simulink library "qss_tb_library_aalto"  (Simulink 8.3)
settings: Solver=ode45  SolverMode=SingleTasking  StartTime=0.0  StopTime=1220  RelTol=1e-3
undefined symbols (not defined in the file): c_BT_E1, c_BT_E2, c_BT_E3, c_BT_E4, c_BT_L1, c_BT_L2, c_BT_L3, c_BT_L4, cap_BT, cc_done, delta_h_C_air, DiscIntNeverNeededParam, dw_GG_c, eff_FC_max, eta_EG_map, eta_EM_map, g, h, H_o_m, H_u, I_BT_max, i_FC_in, i_FC_max, k1, k2, k3, k4, k_cs, M_air, manual_gearbox, P_CVT_opt, power_max, Q_BT_0, Q_BT_IC, Q_BT_min, Q_SC_IC, r_wheel, rchg_map_BT, rdis_map_BT, rho, rho_f, soc_map_BT, t_c, T_CE_max, T_EG_c, T_EG_max, T_EM_max, T_z, U_BT_0, V, V_CE_map, V_FC_out, voc_map_BT, w_CE_max, w_CE_upper, w_CVT_opt, w_EG_row, w_EG_upper, w_EM_row, w_EM_upper ... (+1)
libraries: simulink x4
(part 1 of 4)
settings Model: Creator=buehli  LastModifiedBy=alajunen  ExtModeAutoUpdateStatusClock=off

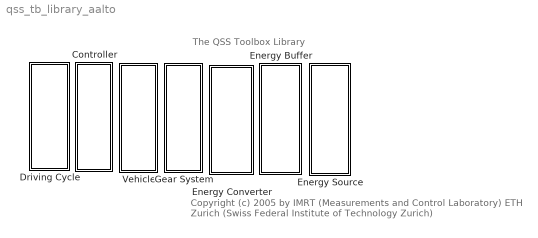
== system qss_tb_library_aalto ==
  note: Copyright (c) 2005 by IMRT (Measurements and Control Laboratory)
      | ETH Zurich (Swiss Federal Institute of Technology Zurich)
  note: The QSS Toolbox Library
  Controller : Subsystem
      mask Display: disp('Controller')
  Driving Cycle : Subsystem
      mask Display: disp('Driving Cycle')
  Energy Buffer : Subsystem
      mask Display: disp('Energy Buffer')
  Energy Converter : Subsystem
      mask Display: disp('Energy Converter')
  Energy Source : Subsystem
      mask Display: disp('Energy Source')
  Gear System : Subsystem
      mask Display: disp('Gear System')
  Vehicle : Subsystem
      mask Display: disp('Vehicle')

== system qss_tb_library_aalto/Controller ==
  Battery Controller : Subsystem  mask(Battery Controller){}
      mask help:
      | Control strategy (very primitive):
      | ========================
      | As soon as battery charge drops below level Q_BT_min, the CE/Generator
      | are started and operated at given load/speed for a fixed time period.
      | This time has been selected to guarantee the same battery level at the
      | end of the cycle.
      mask init:
      | init_BT_ctrl;
  CVT Controller : Subsystem  Tag=cvt controller  mask(CVT Controller){j_CVT_min=3, j_CVT_max=15, w_wheel_min=3, w_CVT_idle=100, w_CVT_upper=300}
      mask prompts: j_CVT_min "Lower gear ratio limit [-]"; j_CVT_max "Upper gear ratio limit [-]"; w_wheel_min "Minimum wheel speed [rad/s]"; w_CVT_idle "CVT idle speed [rad/s]"; w_CVT_upper "Maximum CVT speed [rad/s]"
      mask help:
      | This block calculates the optimum gear ratio and its change during one integration step for a CVT.
      |
      | Input:
      | =====
      | 	v		Speed [m/s]
      | 	dv		Acceleration [m/s^2]
      |
      | Output:
      | ======
      | 	v_delay		Speed one step delayed [m/s]
      | 	dv_delay	Acceleration one step delayed [m/s^2]
      | 	j_CVT		Gear ratio [-]
      | 	dj_CVT		Change of gear ratio [1/s]
      mask init:
      | init_CVT_ctrl;
  Control Unit (empty template) : Subsystem  Tag=control unit  mask(Control Unit){}
      mask help:
      | This block gives the user the opportunity to design his/her own control unit.
      |
      | The user can define the inputs and outputs  by himself/herself.
  Gen-set Controller v2 : Subsystem  mask(Engine-Generator Controller){}
      mask help:
      | Control strategy description:
      | ==============================
      | This block controls the use of the Engine-Generator set (Gen-set).
      | The control system has two different parts: Engine start up/shut down control,
      | and the control of Gen-set power when running.
      |
      | The Engine start up/shut down and Gen-set power are controller by simple rules
      | based on:
      | * vehicle speed, and
      | * battery state-of-charge (soc)
      |
      | The parameters for the Engine start up/shut down control are given in the mask
      | of the block. The parameters for the Gen-set power control are defined in the
      | Look-up tables and the reference control speed is given through the block mask.
      mask init:
      | global h
  Gen-set Controller : Subsystem  mask(Engine-Generator Controller){}
      mask help:
      | Control strategy description:
      | ==============================
      | This block controls the use of the Engine-Generator set (Gen-set).
      | The control system has two different parts: Engine start up/shut down control,
      | and the control of Gen-set power when running.
      |
      | The Engine start up/shut down and Gen-set power are controller by simple rules
      | based on:
      | * vehicle speed, and
      | * battery state-of-charge (soc)
      |
      | The parameters for the Engine start up/shut down control are given in the mask
      | of the block. The parameters for the Gen-set power control are defined in the
      | Look-up tables and the reference control speed is given through the block mask.
      mask init:
      | global h

== system qss_tb_library_aalto/Driving Cycle ==
  Driving Cycle : Subsystem  Tag=cycle  mask(Driving Cycle){cyclenr=Europe: NEDC, stepsize=1, autostop=on}
      mask prompts: cyclenr "Choose a cycle"; stepsize "Step size [s]"; autostop "Enable automatic simulation stop"
      mask help:
      | This block loads the cycle data such as time, speed, acceleration and gear number,  from the specified data file and makes it available on the output of the cycle block.
      |
      | Output:
      | ======
      | 	v	Speed [m/s]
      | 	dv	Acceleration [m/s^2]
      | 	i	Gear number [-]
      | 	x_tot	Total distance [m]
      |
      | Tip:
      | ===
      | Probably you don't need the gear number "i". If so you can terminate
      | it with a "Terminator" out of the "Simulink Library/Connections."
      |
      | Step size:
      | ========
      | Default value is 1. Don't change it, unless you are familiar with the programs of the QSS TB.
      |
      | Enable automatic simulation stop:
      | ===========================
      | Stops the simulation automatically at the end of the cycle.
      | Be careful: If you have a component in your model that has to run after the cycle has finished, e.g. a battery to charge, remove the mark!
      mask init:
      | init_driving_cycle;
      mask TypeOptions cyclenr: Europe: ECE manual | Europe: ECE R15 spez | Europe: ECE R15 | Europe: EUDC | Europe: EUDC manual | Europe: City | Europe: City manual | Europe: NEDC | Europe: NEDC manual | Japan:  10-15-Mode | Japan:  10-Mode | Japan:  10-Mode-3 | Japan:  11-Mode | Japan:  11-Mode-4 | Japan:  15-Mode | USA:    City-I | USA:    City-II | USA:    FTP-75 | USA:    FTP-Highway
      mask Display: plot(T_zplot, V_zplot);
  Driving Cycle v2 : Subsystem  Tag=cycle  mask(Driving Cycle){cyclenr=Europe: NEDC, stepsize=1, autostop=on}
      mask prompts: cyclenr "Choose a cycle"; stepsize "Step size [s]"; autostop "Enable automatic simulation stop"
      mask help:
      | This block loads the cycle data such as time, speed, acceleration and gear number,  from the specified data file and makes it available on the output of the cycle block.
      |
      | Output:
      | ======
      | 	v	Speed [m/s]
      | 	dv	Acceleration [m/s^2]
      | 	i	Gear number [-]
      | 	x_tot	Total distance [m]
      |
      | Tip:
      | ===
      | Probably you don't need the gear number "i". If so you can terminate
      | it with a "Terminator" out of the "Simulink Library/Connections."
      |
      | Step size:
      | ========
      | Default value is 1. Don't change it, unless you are familiar with the programs of the QSS TB.
      |
      | Enable automatic simulation stop:
      | ===========================
      | Stops the simulation automatically at the end of the cycle.
      | Be careful: If you have a component in your model that has to run after the cycle has finished, e.g. a battery to charge, remove the mark!
      mask init:
      | init_driving_cycle_v2;
      mask TypeOptions cyclenr: Europe: ECE manual | Europe: ECE R15 spez | Europe: ECE R15 | Europe: EUDC | Europe: EUDC manual | Europe: City | Europe: City manual | Europe: NEDC | Europe: NEDC manual | Japan:  10-15-Mode | Japan:  10-Mode | Japan:  10-Mode-3 | Japan:  11-Mode | Japan:  11-Mode-4 | Japan:  15-Mode | USA:    City-I | USA:    City-II | USA:    FTP-75 | USA:    FTP-Highway | USA:    US06 | USA:    SC03
      mask Display: plot(T_zplot, V_zplot);
  Driving Cycle v3 : Subsystem  Tag=cycle  mask(Driving Cycle){cyclenr=Europe: NEDC, stepsize=1, autostop=on}
      mask prompts: cyclenr "Choose a cycle"; stepsize "Step size [s]"; autostop "Enable automatic simulation stop"
      mask help:
      | This block loads the cycle data such as time, speed, acceleration and gear number,  from the specified data file and makes it available on the output of the cycle block.
      |
      | Output:
      | ======
      | 	v	Speed [m/s]
      | 	dv	Acceleration [m/s^2]
      | 	i	Gear number [-]
      | 	x_tot	Total distance [m]
      |
      | Tip:
      | ===
      | Probably you don't need the gear number "i". If so you can terminate
      | it with a "Terminator" out of the "Simulink Library/Connections."
      |
      | Step size:
      | ========
      | Default value is 1. Don't change it, unless you are familiar with the programs of the QSS TB.
      |
      | Enable automatic simulation stop:
      | ===========================
      | Stops the simulation automatically at the end of the cycle.
      | Be careful: If you have a component in your model that has to run after the cycle has finished, e.g. a battery to charge, remove the mark!
      mask init:
      | init_driving_cycle_v3;
      mask TypeOptions cyclenr: Europe: ECE manual | Europe: ECE R15 spez | Europe: ECE R15 | Europe: EUDC | Europe: EUDC manual | Europe: City | Europe: City manual | Europe: NEDC | Europe: NEDC manual | Japan:  10-15-Mode | Japan:  10-Mode | Japan:  10-Mode-3 | Japan:  11-Mode | Japan:  11-Mode-4 | Japan:  15-Mode | Japan:  JC08 | USA:    City-I | USA:    City-II | USA:    FTP-75 | USA:    FTP-Highway | USA:    US06 | USA:    SC03 | World:  WLTC
      mask Display: plot(T_zplot, V_zplot);

== system qss_tb_library_aalto/Energy Buffer ==
  Battery : Subsystem  Tag=battery  mask(Battery){I_0=100, Q_BT_IC_rel=27.78, t_ch=20}
      mask prompts: I_0 "Energy capacity of battery [Ah]"; Q_BT_IC_rel "Initial charge of battery [%]"; t_ch "Current limit: minimum time to charge/discharge the battery [min]"
      mask help:
      | This block simulates a battery.
      | The resistance depends on the charge state and the charge/discharge current of the battery. The battery has an open circuit voltage of 130 V (fully charged).
      |
      | Input:
      | =====
      | 	x_tot	Total distance [m]
      | 	P_BT	Power from/to the battery [W]
      | 		P_BT < 0: battery charging
      | 		P_BT > 0: battery discharging
      |
      | Output:
      | ======
      | 	Q_BT	Current charge of the battery [C]
      | 	V_BT	Energy consumption [kWh/100 km]
      mask init:
      | init_BT;
  Battery v2 : Subsystem  Tag=battery  mask(Battery){init_soc_BT=0.7, cell_series_BT=70, cell_parallel_BT=1, init_file_BT='init_Saft_BT'}
      mask prompts: init_soc_BT "Initial charge of battery"; cell_series_BT "Cells in series"; cell_parallel_BT "Cells in parallel"; init_file_BT "Battery initialization file"
      mask init:
      | eval(init_file_BT)
  Battery v3 : Subsystem  Tag=battery  mask(Battery){init_soc_BT=0.7, cell_series_BT=70, cell_parallel_BT=1, init_file_BT='init_Saft_BT'}
      mask prompts: init_soc_BT "Initial charge of battery"; cell_series_BT "Cells in series"; cell_parallel_BT "Cells in parallel"; init_file_BT "Battery initialization file"
      mask init:
      | eval(init_file_BT)
  Supercapacitor : Subsystem  Tag=supercap  mask(Supercapacitor){C_SC=8, R_SC=0.72, U_SC_max=225, P_SC_max=17500, Q_SC_IC_rel=95, N_SC=6}
      mask prompts: C_SC "Capacity of each supercap [F]"; R_SC "Internal resistance of each supercap [Ohm]"; U_SC_max "Maximum voltage of each supercap  [V]"; P_SC_max "Maximum power of each supercap [W]"; Q_SC_IC_rel "Initial charge of each supercap [%]"; N_SC "Number of supercaps (parallel connection) [-]"
      mask help:
      | The supercap is a fast electric energy buffer.
      |
      | Input:
      | =====
      | 	P_SC	Power to/from the supercap [W]
      | 		P_SC < 0: SC charging
      | 		P_SC > 0: SC discharging
      |
      | Output:
      | ======
      | 	U_SC	Voltage of the supercap [V]
      mask init:
      | init_SC;
  Supercapacitor v2 : Subsystem  Tag=supercap  mask(Supercapacitor){C_SC=8, R_SC=0.72, U_SC_max=225, P_SC_max=17500, Q_SC_IC_rel=90, N_SC=6}
      mask prompts: C_SC "Capacity of each supercap [F]"; R_SC "Internal resistance of each supercap [Ohm]"; U_SC_max "Maximum voltage of each supercap  [V]"; P_SC_max "Maximum power of each supercap [W]"; Q_SC_IC_rel "Initial charge of each supercap [%]"; N_SC "Number of supercaps (parallel connection) [-]"
      mask help:
      | The supercap is a fast electric energy buffer.
      |
      | Input:
      | =====
      | 	P_SC	Power to/from the supercap [W]
      | 		P_SC < 0: SC charging
      | 		P_SC > 0: SC discharging
      |
      | Output:
      | ======
      | 	U_SC	Voltage of the supercap [V]
      mask init:
      | init_SC_hyb;
  Supercapacitor v3 : Subsystem  Tag=supercap  mask(Supercapacitor){C_SC=8, R_SC=0.72, U_SC_max=225, P_SC_max=17500, Q_SC_IC_rel=80, N_SC=6}
      mask prompts: C_SC "Capacity of each supercap [F]"; R_SC "Internal resistance of each supercap [Ohm]"; U_SC_max "Maximum voltage of each supercap  [V]"; P_SC_max "Maximum power of each supercap [W]"; Q_SC_IC_rel "Initial charge of each supercap [%]"; N_SC "Number of supercaps (parallel connection) [-]"
      mask help:
      | The supercap is a fast electric energy buffer.
      |
      | Input:
      | =====
      | 	P_SC	Power to/from the supercap [W]
      | 		P_SC < 0: SC charging
      | 		P_SC > 0: SC discharging
      |
      | Output:
      | ======
      | 	U_SC	Voltage of the supercap [V]
      mask init:
      | init_SC_hyb_v2;

== system qss_tb_library_aalto/Energy Converter ==
  Combustion Engine (Willans-approximation) : Subsystem  Tag=combustion engine  mask(Combustion Engine (based on Willans approximation)){engine_type=Otto, V_d=0.708, theta_CE=0.05, S=50, B=45, w_CE_idle=105, P_CE_idle=2600, P_aux=300, e=0.46, PI=2, p_me0g=1, ENABLE_FUEL_CUTOFF=on, T_CE_cutoff=5, P_CE_cutoff=0}
      mask prompts: engine_type "Engine type"; V_d "Displacement [l]"; theta_CE "Engine inertia [kg*m^2]"; S "Stroke [mm]"; B "Bore diameter [mm]"; w_CE_idle "Engine speed at idle [rad/s]"; P_CE_idle "Engine power at idle [W]"; P_aux "Power required by auxiliaries  [W]"; e "1. Willans parameter: Engine internal thermodynamic efficiency [-]"; PI "2. Willans parameter: Maximum boost ratio [-]"; p_me0g "3. Willans parameter: Gas exchange losses [bar]"; ENABLE_FUEL_CUTOFF "Enable fuel cutoff"; T_CE_cutoff "Engine torque at fuel cutoff [Nm]"; P_CE_cutoff "Power at fuel cutoff [W]"
      mask help:
      | This block simulates the behaviour of a combustion engine. The block is based on the Willans approximation with friction part based on the ETH model.
      |
      | Input:
      | =====
      | 	w_gear		Speed of the fly wheel [rad/s]
      | 	dw_gear	Acceleration of the fly wheel [rad/s^2]
      | 	T_gear		Torque on the fly wheel [Nm]
      |
      | Output:
      | ======
      | 	P_CE		Power produced by the combustion engine [W]
      mask init:
      | init_CE_willans;
      mask TypeOptions engine_type: Otto | Diesel
  Combustion Engine (consumption map) : Subsystem  Tag=combustion engine  mask(Combustion Engine (based on consumption map)){engine_type=Otto, V_d=0.708, scale_CE=1, theta_CE=0.05, w_CE_idle=105, P_CE_idle=2600, P_aux=300, ENABLE_FUEL_CUTOFF=on, T_CE_cutoff=5, P_CE_cutoff=0}
      mask prompts: engine_type "Engine type"; V_d "Displacement [l]"; scale_CE "Engine scaling factor [-]"; theta_CE "Engine inertia [kg*m^2]"; w_CE_idle "Engine speed at idle [rad/s]"; P_CE_idle "Engine power at idle [W]"; P_aux "Power required by auxiliaries [W]"; ENABLE_FUEL_CUTOFF "Enable fuel cutoff"; T_CE_cutoff "Engine torque at fuel cutoff [Nm]"; P_CE_cutoff "Power at fuel cutoff [W]"
      mask help:
      | This block simulates the behaviour of a combustion engine. The block is based on a consumption map.
      |
      | Input:
      | =====
      | 	w_gear		Speed of the fly wheel [rad/s]
      | 	dw_gear	Acceleration of the fly wheel [rad/s^2]
      | 	T_gear		Torque on the fly wheel [Nm]
      |
      | Output:
      | ======
      | 	P_CE		Power produced by the combustion engine [W]
      mask init:
      | init_CE_map;
      mask TypeOptions engine_type: Otto | Diesel
  Combustion Engine (hybrid vehicle) : Subsystem  Tag=combustion engine  mask(Combustion Engine (based on consumption map)){engine_type=Otto, V_d=1.0, theta_CE=0.05, w_CE_idle=105, P_CE_idle=0, P_aux=0, ENABLE_FUEL_CUTOFF=on, T_CE_cutoff=0, P_CE_cutoff=0}
      mask prompts: engine_type "Engine type"; V_d "Displacement [l]"; theta_CE "Engine inertia [kg*m^2]"; w_CE_idle "Engine speed at idle [rad/s]"; P_CE_idle "Engine power at idle [W]"; P_aux "Power required by auxiliaries [W]"; ENABLE_FUEL_CUTOFF "Enable fuel cutoff"; T_CE_cutoff "Engine torque at fuel cutoff [Nm]"; P_CE_cutoff "Power at fuel cutoff [W]"
      mask help:
      | This block simulates the behaviour of a combustion engine. The block is based on a consumption map.
      |
      | Input:
      | =====
      | 	w_gear		Speed of the fly wheel [rad/s]
      | 	dw_gear	Acceleration of the fly wheel [rad/s^2]
      | 	T_gear		Torque on the fly wheel [Nm]
      |
      | Output:
      | ======
      | 	P_CE		Power produced by the combustion engine [W]
      mask init:
      | init_CE_hyb_map;
      mask TypeOptions engine_type: Otto
  Combustion Engine (hybrid vehicle) v2 : Subsystem  Tag=combustion engine  mask(Combustion Engine (based on consumption map)){engine_type=Otto, V_d=V, theta_CE=0.16, w_CE_idle=105, P_CE_idle=0, P_aux=0, ENABLE_FUEL_CUTOFF=on, T_CE_cutoff=0, P_CE_cutoff=0}
      mask prompts: engine_type "Engine type"; V_d "Displacement [l]"; theta_CE "Engine inertia [kg*m^2]"; w_CE_idle "Engine speed at idle [rad/s]"; P_CE_idle "Engine power at idle [W]"; P_aux "Power required by auxiliaries [W]"; ENABLE_FUEL_CUTOFF "Enable fuel cutoff"; T_CE_cutoff "Engine torque at fuel cutoff [Nm]"; P_CE_cutoff "Power at fuel cutoff [W]"
      mask help:
      | This block simulates the behaviour of a combustion engine. The block is based on a consumption map.
      |
      | Input:
      | =====
      | w_gear	Speed of the fly wheel [rad/s]
      | dw_gear	Acceleration of the fly wheel [rad/s^2]
      | T_gear	Torque on the fly wheel [Nm]
      |
      | Output:
      | ======
      | P_CE	Power produced by the combustion engine [W]
      mask init:
      | init_CE_Prius_map;
      mask TypeOptions engine_type: Otto
  Combustion Engine v2 : Subsystem  Tag=combustion engine  mask(Combustion Engine (based on consumption map)){engine_type=Otto, V_d=1.9, theta_CE=0.1, w_CE_idle=105, P_CE_idle=2600, P_aux=300, ENABLE_FUEL_CUTOFF=on, T_CE_cutoff=5, P_CE_cutoff=0}
      mask prompts: engine_type "Engine type"; V_d "Displacement [l]"; theta_CE "Engine inertia [kg*m^2]"; w_CE_idle "Engine speed at idle [rad/s]"; P_CE_idle "Engine power at idle [W]"; P_aux "Power required by auxiliaries [W]"; ENABLE_FUEL_CUTOFF "Enable fuel cutoff"; T_CE_cutoff "Engine torque at fuel cutoff [Nm]"; P_CE_cutoff "Power at fuel cutoff [W]"
      mask help:
      | This block simulates the behaviour of a combustion engine. The block is based on a consumption map.
      |
      | Input:
      | =====
      | 	w_gear		Speed of the fly wheel [rad/s]
      | 	dw_gear	Acceleration of the fly wheel [rad/s^2]
      | 	T_gear		Torque on the fly wheel [Nm]
      |
      | Output:
      | ======
      | 	P_CE		Power produced by the combustion engine [W]
      mask init:
      | % Spark ignited (SI)
      | if engine_type == 1
      |     init_SI_CE_map;
      | end
      | % Compression ignited (CI)
      | if engine_type == 2
      |     init_CI_CE_map;
      | end
      mask TypeOptions engine_type: Otto | Diesel
  Combustion Engine v3 : Subsystem  Tag=combustion engine  mask(Combustion Engine (based on consumption map)){engine_type=Otto, V_d=1.9, theta_CE=0.1, w_CE_idle=105, P_CE_idle=0, P_aux=300, ENABLE_FUEL_CUTOFF=on, T_CE_cutoff=2, P_CE_cutoff=0}
      mask prompts: engine_type "Engine type"; V_d "Displacement [l]"; theta_CE "Engine inertia [kg*m^2]"; w_CE_idle "Engine speed at idle [rad/s]"; P_CE_idle "Engine power at idle [W]"; P_aux "Power required by auxiliaries [W]"; ENABLE_FUEL_CUTOFF "Enable fuel cutoff"; T_CE_cutoff "Engine torque at fuel cutoff [Nm]"; P_CE_cutoff "Power at fuel cutoff [W]"
      mask help:
      | This block simulates the behaviour of a combustion engine. The block is based on a consumption map.
      |
      | Input:
      | =====
      | w_gear	Speed of the fly wheel [rad/s]
      | dw_gear	Acceleration of the fly wheel [rad/s^2]
      | T_gear	Torque on the fly wheel [Nm]
      |
      | Output:
      | ======
      | P_CE	Power produced by the combustion engine [W]
      mask init:
      | % Spark ignited (SI)
      | if engine_type == 1
      |     init_SI_CE_map_v2;
      | end
      | % Compression ignited (CI)
      | if engine_type == 2
      |     init_CI_CE_map_v2;
      | end
      mask TypeOptions engine_type: Otto | Diesel
  Electric Generator : Subsystem  mask(Electric Generator){scale_EG=1}
      mask prompts: scale_EG "Generator scaling factor [-]"
      mask help:
      | This block simulates the behaviour of an electric generator. The block is based on an efficiency map.
      |
      | Input:
      | =====
      | 	w_gear		Speed of the fly wheel [rad/s]
      | 	T_gear		Torque on the fly wheel [Nm]
      |
      | Output:
      | ======
      | 	P_EG		Power of the electric generator [W]
      mask init:
      | init_EG;
  Electric Generator v2 : Subsystem  mask(Electric Generator){}
      mask help:
      | This block simulates the behaviour of an electric generator. The block is based on an efficiency map.
      |
      | Input:
      | =====
      | 	w_gear		Speed of the fly wheel [rad/s]
      | 	T_gear		Torque on the fly wheel [Nm]
      |
      | Output:
      | ======
      | 	P_EG		Power of the electric generator [W]
      mask init:
      | init_EG_hyb;
  Electric Generator v3 : Subsystem  mask(Electric Generator){init_file_name='init_EG_UQM'}
      mask prompts: init_file_name "Initialization file name"
      mask help:
      | This block simulates the behaviour of an electric generator. The block is based on an efficiency map.
      |
      | Input:
      | =====
      | w_gear		Speed of the transmission [rad/s]
      | T_gear		Torque of the transmission [Nm]
      |
      | Output:
      | ======
      | P_EG		Power of the electric generator [W]
      mask init:
      | eval(init_file_name);
  Electric Motor : Subsystem  mask(Electric Motor){scale_EM=1, theta_EM=0.1, P_aux=0}
      mask prompts: scale_EM "Motor scaling factor [-]"; theta_EM "Motor inertia [kg*m2]"; P_aux "Power required by auxiliaries [W]"
      mask help:
      | This block simulates the behaviour of an electric motor. The block is based on an efficiency map.
      |
      | Input:
      | =====
      | 	w_gear		Speed of the fly wheel [rad/s]
      | 	dw_gear	Acceleration of the fly wheel [rad/s^2]
      | 	T_gear		Torque on the fly wheel [Nm]
      |
      | Output:
      | ======
      | 	P_EM		Power produced by the electric motor [W]
      mask init:
      | init_EM;
  Electric Motor v2 : Subsystem  mask(Electric Motor){scale_EM=3.5, theta_EM=0.1, P_aux=300, over_factor=1.25}
      mask prompts: scale_EM "Motor scaling factor [-]"; theta_EM "Motor inertia [kg*m2]"; P_aux "Power required by auxiliaries [W]"; over_factor "Overtorque factor"
      mask help:
      | This block simulates the behaviour of an electric motor. The block is based on an efficiency map.
      |
      | Input:
      | =====
      | 	w_gear		Speed of the fly wheel [rad/s]
      | 	dw_gear	Acceleration of the fly wheel [rad/s^2]
      | 	T_gear		Torque on the fly wheel [Nm]
      |
      | Output:
      | ======
      | 	P_EM		Power produced by the electric motor [W]
      mask init:
      | init_EM;
  Fuel Cell : Subsystem  Tag=fuelcell  mask(Fuel Cell){N_FC=880, A_FC=190 * 1e4, V_th=1.2, P_FC_idle=2000, eta_EM_C=0.75, eta_C=0.7, pi_C=1.3, T_air=25, l_air=1.5}
      mask prompts: N_FC "Number of fuel cells per stack (series connection) [-]"; A_FC "Size of fuel cell [m^2]"; V_th "Theoretical fuel cell voltage [V]"; P_FC_idle "Idle power [W]"; eta_EM_C "E-motor for air compressor efficiency [-]"; eta_C "Air compressor efficiency [-]"; pi_C "Air compression ratio [-]"; T_air "Air temperature [°C]"; l_air "Air to fuel ratio [-]"
      mask help:
      | This block simulates a fuel cell and converts fuel into electric energy.
      |
      | Input:
      | =====
      | 	P_in		Power required by the fuel cell [W]
      |
      | Output:
      | ======
      | 	P_FC		Power produced by the fuel cell [W]
      mask init:
      | init_FC;
  Fuel Cell v2 : Subsystem  Tag=fuelcell  mask(Fuel Cell){N_FC=120, A_FC=0.084, V_th=1.2, P_FC_idle=2000, eta_EM_C=0.75, eta_C=0.7, pi_C=1.3, T_air=25, l_air=1.5}
      mask prompts: N_FC "Number of fuel cells per stack (series connection) [-]"; A_FC "Size of a single fuel cell [m^2]"; V_th "Theoretical fuel cell voltage [V]"; P_FC_idle "Idle power [W]"; eta_EM_C "E-motor for air compressor efficiency [-]"; eta_C "Air compressor efficiency [-]"; pi_C "Air compression ratio [-]"; T_air "Air temperature [°C]"; l_air "Air to fuel ratio [-]"
      mask help:
      | This block simulates a fuel cell and converts fuel into electric energy.
      |
      | Input:
      | =====
      | 	P_in		Power required by the fuel cell [W]
      |
      | Output:
      | ======
      | 	P_FC		Power produced by the fuel cell [W]
      mask init:
      | init_FC_hyb;

== system qss_tb_library_aalto/Energy Source ==
  Display : Display
  Hydrogen Tank : Subsystem  Tag=tank  mask(Tank){flag_cold_start=off}
      mask prompts: flag_cold_start "Include cold start losses"
      mask help:
      | This block integrates the power (the fuel mass flow) required by the combustion engine or the fuel cell and calculates the energy consumption in liter/100 km.
      |
      | Input:
      | =====
      | 	P_fuel	Power (fuel mass flow) required [W]
      | 	x_tot	Total distance [m]
      |
      | Output:
      | ======
      | 	V	Fuel consumption [liter/100 km]
      mask init:
      | init_tank_v2;
  Tank : Subsystem  Tag=tank  mask(Tank){fuel=Gasoline, flag_cold_start=on}
      mask prompts: flag_cold_start "Include cold start losses"
      mask help:
      | This block integrates the power (the fuel mass flow) required by the combustion engine or the fuel cell and calculates the energy consumption in liter/100 km.
      |
      | Input:
      | =====
      | 	P_fuel	Power (fuel mass flow) required [W]
      | 	x_tot	Total distance [m]
      |
      | Output:
      | ======
      | 	V	Fuel consumption [liter/100 km]
      mask init:
      | init_tank;
      mask TypeOptions fuel: Gasoline | Diesel | Hydrogen
  Tank v2 : Subsystem  Tag=tank  mask(Tank){flag_cold_start=off}
      mask prompts: flag_cold_start "Include cold start losses"
      mask help:
      | This block integrates the power (the fuel mass flow) required by the combustion engine or the fuel cell and calculates the energy consumption in liter/100 km.
      |
      | Input:
      | =====
      | 	P_fuel	Power (fuel mass flow) required [W]
      | 	x_tot	Total distance [m]
      |
      | Output:
      | ======
      | 	V	Fuel consumption [liter/100 km]
      mask init:
      | init_tank_v2;
  kg/100km hydrogen : Display
  liters/100km : Display
  liters/100km gasoline equivalent : Display
  wires:
  Tank/1(liter/100 km) -> Display/1
  Hydrogen Tank/1(kg/100 km) -> kg/100km hydrogen/1
  Hydrogen Tank/2(liter/100 km) -> liters/100km gasoline equivalent/1
  Tank v2/1(liter/100 km) -> liters/100km/1

== system qss_tb_library_aalto/Gear System ==
  Continuously Variable Transmission : Subsystem  Tag=cvt  mask(CVT){e_CVT=0.97, P_CVT0=400, w_wheel_min=3}
      mask prompts: e_CVT "Efficiency [-]"; P_CVT0 "Idling losses (friction) [W]"; w_wheel_min "Minimum wheel speed beyond which losses are generated [rad/s]"
      mask help:
      | This block simulates a CVT transmission.
      |
      | Input:
      | =====
      | 	w_wheel	Speed of the wheel [rad/s]
      | 	dw_wheel	Acceleration of the wheel [rad/s^2],
      | 	T_wheel	Torque on the wheel [Nm]
      | 	j_CVT		Gear ratio [-]
      | 	dj_CVT		Change of gear ratio [1/s]
      |
      | Output:
      | ======
      | 	w_CVT		Speed of the fly wheel [rad/s]
      | 	dw_CVT	Acceleration of the fly wheel [rad/s^2]
      | 	T_CVT		Torque on the fly wheel [Nm]
      mask init:
      | init_CVT;
  Manual Gear Box : Subsystem  Tag=transmission  mask(Manual Gear Box){i_1=15.174, i_2=8.338, i_3=5.378, i_4=3.937, i_5=2.748, i_diff=1, e_GT=0.98, P_GT0=300, w_wheel_min=1}
      mask prompts: i_1 "1. gear [-]"; i_2 "2. gear [-]"; i_3 "3. gear [-]"; i_4 "4. gear [-]"; i_5 "5. gear [-]"; i_diff "Differential gear [-]"; e_GT "Efficiency [-]"; P_GT0 "Idling losses (friction) [W]"; w_wheel_min "Minimum wheel speed beyond which losses are generated [rad/s]"
      mask help:
      | This block simulates a manual gear box.
      |
      | Input:
      | =====
      | 	w_wheel	Speed of the wheel [rad/s]
      | 	dw_wheel	Acceleration of the wheel [rad/s^2],
      | 	T_wheel	Torque on the wheel [Nm]
      | 	i		Gear number [-]
      |
      | Output:
      | ======
      | 	w_MGB		Speed of the fly wheel [rad/s]
      | 	dw_MGB	Acceleration of the fly wheel [rad/s^2]
      | 	T_MGB		Torque on the fly wheel [Nm]
      mask init:
      | init_MGB;
  Simple Transmission : Subsystem  Tag=simple transmission  mask(Simple Transmission){gear_ratio=3, e_GT=0.98, P_GT0=50, w_wheel_min=1}
      mask prompts: gear_ratio "Gear ratio [-]"; e_GT "Efficiency [-]"; P_GT0 "Idling losses (friction) [W]"; w_wheel_min "Minimum wheel speed beyond which losses are generated [rad/s]"
      mask help:
      | This block simulates a transmission with a fixed gear ratio.
      |
      | Input:
      | =====
      | 	w_wheel	Speed of the wheel [rad/s]
      | 	dw_wheel	Acceleration of the wheel [rad/s^2]
      | 	T_wheel	Torque on the wheel [Nm]
      |
      | Output:
      | ======
      | 	w_trans		Speed of the fly wheel [rad/s]
      | 	dw_trans	Acceleration of the fly wheel [rad/s^2]
      | 	T_trans		Torque on the fly wheel [Nm]
      mask init:
      | init_transmission;
  Transmission CE-EG : Subsystem  Tag=simple transmission  mask(Transmission){gear_ratio=0.75, e_GT=0.98, P_GT0=200, w_wheel_min=0}
      mask prompts: gear_ratio "Gear ratio [-]"; e_GT "Efficiency [-]"; P_GT0 "Idling losses (friction) [W]"; w_wheel_min "Minimum wheel speed beyond which losses are generated [rad/s]"
      mask help:
      | This block simulates a transmission with a fixed gear ratio.
      |
      | Input:
      | =====
      | 	w_wheel	Speed of the wheel [rad/s]
      | 	dw_wheel	Acceleration of the wheel [rad/s^2]
      | 	T_wheel	Torque on the wheel [Nm]
      |
      | Output:
      | ======
      | 	w_trans		Speed of the fly wheel [rad/s]
      | 	dw_trans	Acceleration of the fly wheel [rad/s^2]
      | 	T_trans		Torque on the fly wheel [Nm]
      mask init:
      | init_transmission;
  Transmission CE-EG v2 : Subsystem  Tag=simple transmission  mask(Transmission){gear_ratio=1.6, e_GT=0.98, P_GT0=200, w_wheel_min=0}
      mask prompts: gear_ratio "Gear ratio [-]"; e_GT "Efficiency [-]"; P_GT0 "Idling losses (friction) [W]"; w_wheel_min "Minimum wheel speed beyond which losses are generated [rad/s]"
      mask help:
      | This block simulates a transmission with a fixed gear ratio.
      |
      | Input:
      | =====
      | w_CE        Speed of the engine [rad/s]
      | dw_CE       Acceleration of the engine [rad/s^2]
      | T_CE        Torque of the engine [Nm]
      |
      | Output:
      | ======
      | w_trans     Speed of the transmission [rad/s]
      | dw_trans    Acceleration of the transmission [rad/s^2]
      | T_trans     Torque of the transmission [Nm]
      mask init:
      | init_transmission;
  Transmission Vehicle-EM : Subsystem  Tag=simple transmission  mask(Transmission){gear_ratio=3.5, e_GT=0.98, P_GT0=300, w_wheel_min=1}
      mask prompts: gear_ratio "Gear ratio [-]"; e_GT "Efficiency [-]"; P_GT0 "Idling losses (friction) [W]"; w_wheel_min "Minimum wheel speed beyond which losses are generated [rad/s]"
      mask help:
      | This block simulates a transmission with a fixed gear ratio.
      |
      | Input:
      | =====
      | 	w_wheel	Speed of the wheel [rad/s]
      | 	dw_wheel	Acceleration of the wheel [rad/s^2]
      | 	T_wheel	Torque on the wheel [Nm]
      |
      | Output:
      | ======
      | 	w_trans		Speed of the fly wheel [rad/s]
      | 	dw_trans	Acceleration of the fly wheel [rad/s^2]
      | 	T_trans		Torque on the fly wheel [Nm]
      mask init:
      | init_transmission;

== system qss_tb_library_aalto/Vehicle ==
  Vehicle : Subsystem  Tag=vehicle  mask(Vehicle){m_f=750, mt2m_f=5, A_f=1.8, d_wheel=0.5, cw=0.22, mu=0.008}
      mask prompts: m_f "Total mass of the vehicle [kg]"; mt2m_f "Rotating mass [%]"; A_f "Vehicle cross section [m^2]"; d_wheel "Wheel diameter [m]"; cw "Drag coefficient [-]"; mu "Rolling friction coefficient [-]"
      mask help:
      | This block computes the power required from the vehicle.
      |
      | Input:
      | =====
      | 	v		Speed [m/s]
      | 	dv		Acceleration [m/s^2]
      |
      | Output:
      | ======
      | 	w_wheel	Speed of the wheel [rad/s]
      | 	dw_wheel	Acceleration of the wheel [rad/s^2]
      | 	T_wheel	Torque on the wheel [Nm]
      mask init:
      | init_vehicle;
  Vehicle v2 : Subsystem  Tag=vehicle  mask(Vehicle){m_f=1200, mt2m_f=5, A_f=2.0, d_wheel=0.6, cw=0.33, mu=0.01}
      mask prompts: m_f "Total mass of the vehicle [kg]"; mt2m_f "Rotating mass [%]"; A_f "Vehicle cross section [m^2]"; d_wheel "Wheel diameter [m]"; cw "Drag coefficient [-]"; mu "Rolling friction coefficient [-]"
      mask help:
      | This block computes the power required from the vehicle.
      |
      | Input:
      | =====
      | 	v		Speed [m/s]
      | 	dv		Acceleration [m/s^2]
      |
      | Output:
      | ======
      | 	w_wheel	Speed of the wheel [rad/s]
      | 	dw_wheel	Acceleration of the wheel [rad/s^2]
      | 	T_wheel	Torque on the wheel [Nm]
      mask init:
      | init_vehicle_default_v2;

== system qss_tb_library_aalto/Controller/Battery Controller ==
  Q_BT : Inport
  Constant : Constant  OutDataTypeStr=boolean
  Constant1 : Constant  Value=Q_BT_min
  Constant2 : Constant  Value=0  OutDataTypeStr=boolean
  Demux : Demux  Outputs=3
  Geno-Group On : Subsystem
  S-R Flip-Flop : Subsystem
  Sum : Sum  Inputs=+-  SaturateOnIntegerOverflow=on  InputSameDT=on  OutDataTypeStr=Inherit: Same as first input
  Switch : Switch  SaturateOnIntegerOverflow=on  InputSameDT=on
  Terminator1 : Terminator
  To Workspace1 : ToWorkspace  VariableName=w_ctrl  SampleTime=-1
  To Workspace2 : ToWorkspace  VariableName=T_ctrl  SampleTime=-1
  To Workspace5 : ToWorkspace  VariableName=cc_on  SampleTime=-1
  w_ctrl : Outport  InitialOutput=0
  dw_ctrl : Outport  Port=2  InitialOutput=0
  T_ctrl : Outport  Port=3  InitialOutput=0
  wires:
  S-R Flip-Flop/1(Q) -> To Workspace5/1, Geno-Group On/1(cc_on)
  Switch/1 -> S-R Flip-Flop/1(S)
  S-R Flip-Flop/2(!Q) -> Terminator1/1
  Geno-Group On/1(OutOn) -> Demux/1
  Demux/3 -> To Workspace2/1, T_ctrl/1
  Demux/2 -> dw_ctrl/1
  Demux/1 -> To Workspace1/1, w_ctrl/1
  Geno-Group On/2(done) -> S-R Flip-Flop/2(R)
  Q_BT/1 -> Sum/1
  Sum/1 -> Switch/2
  Constant2/1 -> Switch/1
  Constant/1 -> Switch/3
  Constant1/1 -> Sum/2

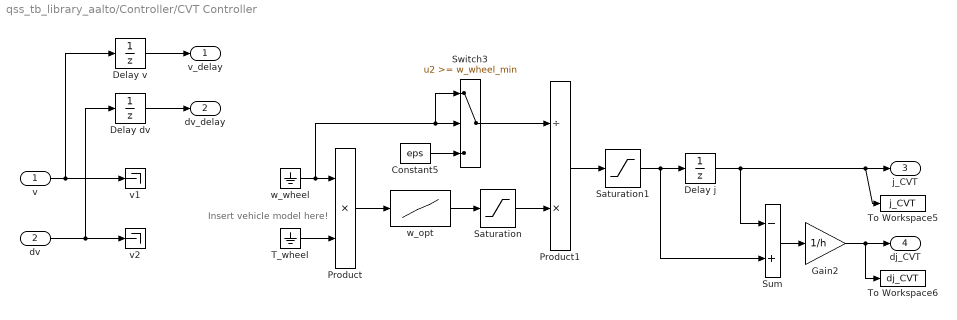
== system qss_tb_library_aalto/Controller/CVT Controller ==
  note: Insert vehicle
      | model here!
  v : Inport
  dv : Inport  Port=2
  Constant5 : Constant  Value=eps
  Delay dv : UnitDelay  SampleTime=h
  Delay j : UnitDelay  InitialCondition=j_CVT_min  SampleTime=h
  Delay v : UnitDelay  SampleTime=h
  Gain2 : Gain  Gain=1/h  SaturateOnIntegerOverflow=on  OutDataTypeStr=Inherit: Same as input  ParamDataTypeStr=Inherit: Same as input
  Product : Product  SaturateOnIntegerOverflow=on  RndMeth=Zero  InputSameDT=on  OutDataTypeStr=Inherit: Same as first input
  Product1 : Product  Inputs=/*  SaturateOnIntegerOverflow=on  RndMeth=Zero  InputSameDT=on  OutDataTypeStr=Inherit: Same as first input
  Saturation : Saturate  UpperLimit=w_CVT_upper  LowerLimit=w_CVT_idle
  Saturation1 : Saturate  UpperLimit=j_CVT_max  LowerLimit=j_CVT_min
  Sum : Sum  Inputs=-+  SaturateOnIntegerOverflow=on  InputSameDT=on  OutDataTypeStr=Inherit: Same as first input
  Switch3 : Switch  Threshold=w_wheel_min  SaturateOnIntegerOverflow=on  InputSameDT=on
  T_wheel : Ground
  To Workspace5 : ToWorkspace  VariableName=j_CVT  SampleTime=-1
  To Workspace6 : ToWorkspace  VariableName=dj_CVT  SampleTime=-1
  v1 : Terminator
  v2 : Terminator
  w_opt : Lookup  InputValues=P_CVT_opt  Table=w_CVT_opt  SaturateOnIntegerOverflow=on
  w_wheel : Ground
  v_delay : Outport  InitialOutput=0
  dv_delay : Outport  Port=2  InitialOutput=0
  j_CVT : Outport  Port=3  InitialOutput=0
  dj_CVT : Outport  Port=4  InitialOutput=0
  wires:
  Gain2/1 -> To Workspace6/1, dj_CVT/1
  T_wheel/1 -> Product/2
  Product1/1 -> Saturation1/1
  Saturation/1 -> Product1/2
  w_wheel/1 -> Switch3/2, Switch3/1, Product/1
  Constant5/1 -> Switch3/3
  dv/1 -> Delay dv/1, v2/1
  v/1 -> Delay v/1, v1/1
  Delay dv/1 -> dv_delay/1
  Switch3/1 -> Product1/1
  Delay j/1 -> To Workspace5/1, j_CVT/1, Sum/1
  Saturation1/1 -> Delay j/1, Sum/2
  Product/1 -> w_opt/1
  w_opt/1 -> Saturation/1
  Delay v/1 -> v_delay/1
  Sum/1 -> Gain2/1

== system qss_tb_library_aalto/Controller/Control Unit (empty template) ==
  note: Control Unit: custom designed
  y 1 : Inport
  y p : Inport  Port=2
  Ground : Ground
  Ground1 : Ground
  Terminator : Terminator
  Terminator1 : Terminator
  u 1 : Outport  InitialOutput=0
  u m : Outport  Port=2  InitialOutput=0
  wires:
  Ground/1 -> u 1/1
  Ground1/1 -> u m/1
  y 1/1 -> Terminator/1
  y p/1 -> Terminator1/1

== system qss_tb_library_aalto/Controller/Gen-set Controller v2 ==
  q_BT : Inport
  v : Inport  Port=2
  P_EM : Inport  Port=3
  Demux : Demux  Outputs=2
  Engine start control : Subsystem  mask{spd_min=30, spd_max=45, soc_min=0.5, soc_max=0.7}
      mask prompts: spd_min "Speed limit low (km/h)"; spd_max "Speed limit high (km/h)"; soc_min "SOC limit low"; soc_max "SOC limit high"
      mask Display: disp('Engine start up /\n shut down control')
  Power control : Subsystem  mask{ctrl_speed=2250, spd_coeff=0.045}
      mask prompts: ctrl_speed "Control speed (rpm)"; spd_coeff "Vehicle speed coefficient"
      mask init:
      | init_EG_ctrl;
      mask Display: disp('Gen-set \n power control')
  ToWS_T_ctrl : ToWorkspace  VariableName=T_ctrl  SampleTime=-1
  ToWS_T_ctrl1 : ToWorkspace  VariableName=ice_on  SampleTime=-1
  ToWS_w_ctrl : ToWorkspace  VariableName=w_ctrl  SampleTime=-1
  w_ctrl : Outport  InitialOutput=0
  T_ctrl : Outport  Port=2  InitialOutput=0
  wires:
  v/1 -> Engine start control/1(speed (m/s)), Power control/2(speed (m/s))
  Power control/1(ctrl cmds) -> Demux/1
  P_EM/1 -> Power control/1(power (W))
  Engine start control/1(engine on) -> ToWS_T_ctrl1/1, Power control/4(engine on)
  Demux/2 -> T_ctrl/1, ToWS_T_ctrl/1
  Demux/1 -> w_ctrl/1, ToWS_w_ctrl/1
  q_BT/1 -> Power control/3(soc), Engine start control/2(soc)

== system qss_tb_library_aalto/Controller/Gen-set Controller ==
  q_BT : Inport
  v : Inport  Port=2
  P_EM : Inport  Port=3
  Demux : Demux  Outputs=2
  Engine start control : Subsystem  mask{spd_min=35, spd_max=42, soc_min=0.55, soc_max=0.8}
      mask prompts: spd_min "Speed limit low (km/h)"; spd_max "Speed limit high (km/h)"; soc_min "SOC limit low"; soc_max "SOC limit high"
      mask Display: disp('Engine start up /\n shut down control')
  Power control : Subsystem  mask{ctrl_speed=3500, spd_coeff=0.045}
      mask prompts: ctrl_speed "Control speed (rpm)"; spd_coeff "Vehicle speed coefficient"
      mask init:
      | global w_CE_row
      | global T_CE_max
      | 
      | power_max = 0.9*interp1(w_CE_row, T_CE_max.*w_CE_row, ctrl_speed*pi/30);
      mask Display: disp('Gen-set \n power control')
  ToWS_T_ctrl : ToWorkspace  VariableName=T_ctrl  SampleTime=-1
  ToWS_T_ctrl1 : ToWorkspace  VariableName=ice_on  SampleTime=-1
  ToWS_w_ctrl : ToWorkspace  VariableName=w_ctrl  SampleTime=-1
  w_ctrl : Outport  InitialOutput=0
  T_ctrl : Outport  Port=2  InitialOutput=0
  wires:
  q_BT/1 -> Engine start control/2(soc), Power control/3(soc)
  Demux/1 -> ToWS_w_ctrl/1, w_ctrl/1
  Demux/2 -> ToWS_T_ctrl/1, T_ctrl/1
  Engine start control/1(engine on) -> Power control/4(engine on), ToWS_T_ctrl1/1
  P_EM/1 -> Power control/1(power (W))
  Power control/1(ctrl cmds) -> Demux/1
  v/1 -> Power control/2(speed (m/s)), Engine start control/1(speed (m/s))

== system qss_tb_library_aalto/Driving Cycle/Driving Cycle ==
  note: Speed
  Clock : Clock
  Cycle data : FromWorkspace  VariableName=[T_z, V_z, D_z, G_z]  SampleTime=h
  Demux : Demux  Outputs=3
  Differentiation : Subsystem
  Integration : Subsystem
  Terminator : Terminator
  Time : Display
  To Workspace1 : ToWorkspace  VariableName=t  SampleTime=-1
  To Workspace2 : ToWorkspace  VariableName=x_tot  SampleTime=-1
  To Workspace4 : ToWorkspace  VariableName=dv  SampleTime=-1
  To Workspace5 : ToWorkspace  VariableName=v  SampleTime=-1
  To Workspace6 : ToWorkspace  VariableName=i  SampleTime=-1
  v : Outport  InitialOutput=0
  dv : Outport  Port=2  InitialOutput=0
  i : Outport  Port=3  InitialOutput=0
  x_tot : Outport  Port=4  InitialOutput=0
  wires:
  Cycle data/1 -> Demux/1
  Differentiation/1(D_z) -> To Workspace4/1, dv/1
  Demux/2 -> Terminator/1
  Demux/1 -> Integration/1(V_z), v/1, To Workspace5/1, Differentiation/1(V_z)
  Integration/1(x_tot) -> x_tot/1, To Workspace2/1
  Demux/3 -> i/1, To Workspace6/1  "Gear ratio"
  Clock/1 -> Time/1, To Workspace1/1

== system qss_tb_library_aalto/Driving Cycle/Driving Cycle v2 ==
  note: Speed
  Clock : Clock
  Constant : Constant  Value=length(T_z)
  Cycle data : FromWorkspace  VariableName=[T_z, V_z, D_z, G_z]  SampleTime=h
  Demux : Demux  Outputs=3
  Differentiation : Subsystem
  Integration : Subsystem
  Terminator : Terminator
  Time : Display
  To Workspace1 : ToWorkspace  VariableName=t  SampleTime=-1
  To Workspace2 : ToWorkspace  VariableName=x_tot  SampleTime=-1
  To Workspace3 : ToWorkspace  VariableName=stop_time  SampleTime=-1
      settings: StopFcn=|
      | if stop_time(end) > t(end)                              disp(' ')
      | disp('WARNING: Simulation stopped before the end of the cycle. Check your model for correct component parameters')
      | disp(' ')
      | end
  To Workspace4 : ToWorkspace  VariableName=dv  SampleTime=-1
  To Workspace5 : ToWorkspace  VariableName=v  SampleTime=-1
  To Workspace6 : ToWorkspace  VariableName=i  SampleTime=-1
  v : Outport  InitialOutput=0
  dv : Outport  Port=2  InitialOutput=0
  i : Outport  Port=3  InitialOutput=0
  x_tot : Outport  Port=4  InitialOutput=0
  wires:
  Clock/1 -> To Workspace1/1, Time/1
  Demux/3 -> To Workspace6/1, i/1  "Gear ratio"
  Integration/1(x_tot) -> To Workspace2/1, x_tot/1
  Demux/1 -> Differentiation/1(V_z), To Workspace5/1, v/1, Integration/1(V_z)
  Demux/2 -> Terminator/1
  Differentiation/1(D_z) -> dv/1, To Workspace4/1
  Cycle data/1 -> Demux/1
  Constant/1 -> To Workspace3/1

== system qss_tb_library_aalto/Driving Cycle/Driving Cycle v3 ==
  note: Speed
  Clock : Clock
  Constant : Constant  Value=length(T_z)
  Cycle data : FromWorkspace  VariableName=[T_z, V_z, D_z, G_z]  SampleTime=h
  Demux : Demux  Outputs=3
  Differentiation : Subsystem
  Integration : Subsystem
  Terminator : Terminator
  Time : Display
  To Workspace1 : ToWorkspace  VariableName=t  SampleTime=-1
  To Workspace2 : ToWorkspace  VariableName=x_tot  SampleTime=-1
  To Workspace3 : ToWorkspace  VariableName=stop_time  SampleTime=-1
      settings: StopFcn=|
      | if stop_time(end) > t(end)                              disp(' ')
      | disp('WARNING: Simulation stopped before the end of the cycle. Check your model for correct component parameters')
      | disp(' ')
      | end
  To Workspace4 : ToWorkspace  VariableName=dv  SampleTime=-1
  To Workspace5 : ToWorkspace  VariableName=v  SampleTime=-1
  To Workspace6 : ToWorkspace  VariableName=i  SampleTime=-1
  v : Outport  InitialOutput=0
  dv : Outport  Port=2  InitialOutput=0
  i : Outport  Port=3  InitialOutput=0
  x_tot : Outport  Port=4  InitialOutput=0
  wires:
  Constant/1 -> To Workspace3/1
  Cycle data/1 -> Demux/1
  Differentiation/1(D_z) -> To Workspace4/1, dv/1
  Demux/2 -> Terminator/1
  Demux/1 -> Integration/1(V_z), v/1, To Workspace5/1, Differentiation/1(V_z)
  Integration/1(x_tot) -> x_tot/1, To Workspace2/1
  Demux/3 -> i/1, To Workspace6/1  "Gear ratio"
  Clock/1 -> Time/1, To Workspace1/1

== system qss_tb_library_aalto/Energy Buffer/Battery ==
  P_BT : Inport
  x_tot : Inport  Port=2
  Battery charge : UnitDelay  InitialCondition=Q_BT_IC  SampleTime=h
  Battery voltage : Subsystem
  Constant : Constant  Value=Q_BT_IC
  Gain : Gain  Gain=h  SaturateOnIntegerOverflow=on  OutDataTypeStr=Inherit: Same as input  ParamDataTypeStr=Inherit: Same as input
  Gain1 : Gain  Gain=U_BT_0/3.6e1  SaturateOnIntegerOverflow=on  OutDataTypeStr=Inherit: Same as input  ParamDataTypeStr=Inherit: Same as input
  Gain4 : Gain  Gain=1/Q_BT_0  SaturateOnIntegerOverflow=on  OutDataTypeStr=Inherit: Same as input  ParamDataTypeStr=Inherit: Same as input
  Product1 : Product  Inputs=*/  SaturateOnIntegerOverflow=on  RndMeth=Zero  InputSameDT=on  OutDataTypeStr=Inherit: Same as first input
  Sum3 : Sum  Inputs=+-  SaturateOnIntegerOverflow=on  InputSameDT=on  OutDataTypeStr=Inherit: Same as first input
  Sum4 : Sum  Inputs=+-  SaturateOnIntegerOverflow=on  InputSameDT=on  OutDataTypeStr=Inherit: Same as first input
  To Workspace1 : ToWorkspace  VariableName=q_BT  SampleTime=-1
  To Workspace2 : ToWorkspace  VariableName=U_BT  SampleTime=-1
  To Workspace3 : ToWorkspace  VariableName=I_BT  SampleTime=-1
  To Workspace4 : ToWorkspace  VariableName=Q_BT  SampleTime=-1
  To Workspace5 : ToWorkspace  VariableName=P_BT  SampleTime=-1
  Q_BT : Outport  InitialOutput=0
  V_BT : Outport  Port=2  InitialOutput=0
  wires:
  Battery voltage/2(I_BT) -> Gain/1, To Workspace3/1
  Constant/1 -> Sum4/1
  Sum3/1 -> Battery charge/1
  Gain/1 -> Sum3/2
  Battery charge/1 -> Sum3/1, Gain4/1, Sum4/2, Battery voltage/1(Q_BT), Q_BT/1, To Workspace4/1
  Battery voltage/1(U_BT) -> To Workspace2/1
  x_tot/1 -> Product1/2
  Gain1/1 -> Product1/1
  Product1/1 -> V_BT/1
  Sum4/1 -> Gain1/1
  Gain4/1 -> To Workspace1/1
  P_BT/1 -> Battery voltage/2(P_BT), To Workspace5/1

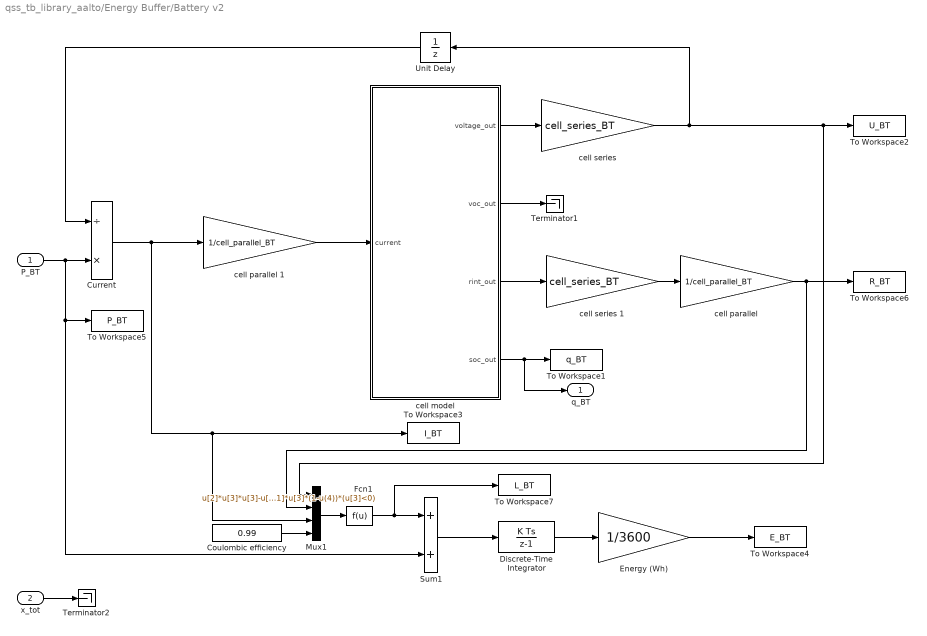
== system qss_tb_library_aalto/Energy Buffer/Battery v2 ==
  P_BT : Inport
  x_tot : Inport  Port=2
  Coulombic efficiency : Constant  Value=0.99
  Current : Product  Inputs=/*  RndMeth=Zero
  Discrete-Time Integrator : DiscreteIntegrator  ICPrevOutput=DiscIntNeverNeededParam  ICPrevScaledInput=DiscIntNeverNeededParam
  Energy (Wh) : Gain  Gain=1/3600
  Fcn1 : Fcn  Expr=u[2]*u[3]*u[3]-u[1]*u[3]*(1-u(4))*(u[3]<0)
  Mux1 : Mux
  Sum1 : Sum  SaturateOnIntegerOverflow=on  InputSameDT=on  OutDataTypeStr=Inherit: Same as first input
  Terminator1 : Terminator
  Terminator2 : Terminator
  To Workspace1 : ToWorkspace  VariableName=q_BT  SampleTime=-1
  To Workspace2 : ToWorkspace  VariableName=U_BT  SampleTime=-1
  To Workspace3 : ToWorkspace  VariableName=I_BT  SampleTime=-1
  To Workspace4 : ToWorkspace  VariableName=E_BT  SampleTime=-1
  To Workspace5 : ToWorkspace  VariableName=P_BT  SampleTime=-1
  To Workspace6 : ToWorkspace  VariableName=R_BT  SampleTime=-1
  To Workspace7 : ToWorkspace  VariableName=L_BT  SampleTime=-1
  Unit Delay : UnitDelay  InitialCondition=cell_series_BT*max(voc_map_BT)  SampleTime=-1
  cell model : Subsystem
  cell parallel : Gain  Gain=1/cell_parallel_BT
  cell parallel 1 : Gain  Gain=1/cell_parallel_BT
  "cell series " : Gain  Gain=cell_series_BT
  cell series 1 : Gain  Gain=cell_series_BT
  q_BT : Outport  InitialOutput=0
  wires:
  cell model/1(voltage_out) -> "cell series "/1
  "cell series "/1 -> Unit Delay/1, To Workspace2/1, Mux1/1
  cell model/3(rint_out) -> cell series 1/1
  cell series 1/1 -> cell parallel/1
  P_BT/1 -> Current/2, To Workspace5/1, Sum1/2
  cell model/2(voc_out) -> Terminator1/1
  Unit Delay/1 -> Current/1
  Current/1 -> cell parallel 1/1, To Workspace3/1, Mux1/3
  cell model/4(soc_out) -> To Workspace1/1, q_BT/1
  cell parallel/1 -> To Workspace6/1, Mux1/2
  cell parallel 1/1 -> cell model/1(current)
  Discrete-Time Integrator/1 -> Energy (Wh)/1
  Fcn1/1 -> Sum1/1, To Workspace7/1
  Sum1/1 -> Discrete-Time Integrator/1
  Energy (Wh)/1 -> To Workspace4/1
  x_tot/1 -> Terminator2/1
  Mux1/1 -> Fcn1/1
  Coulombic efficiency/1 -> Mux1/4

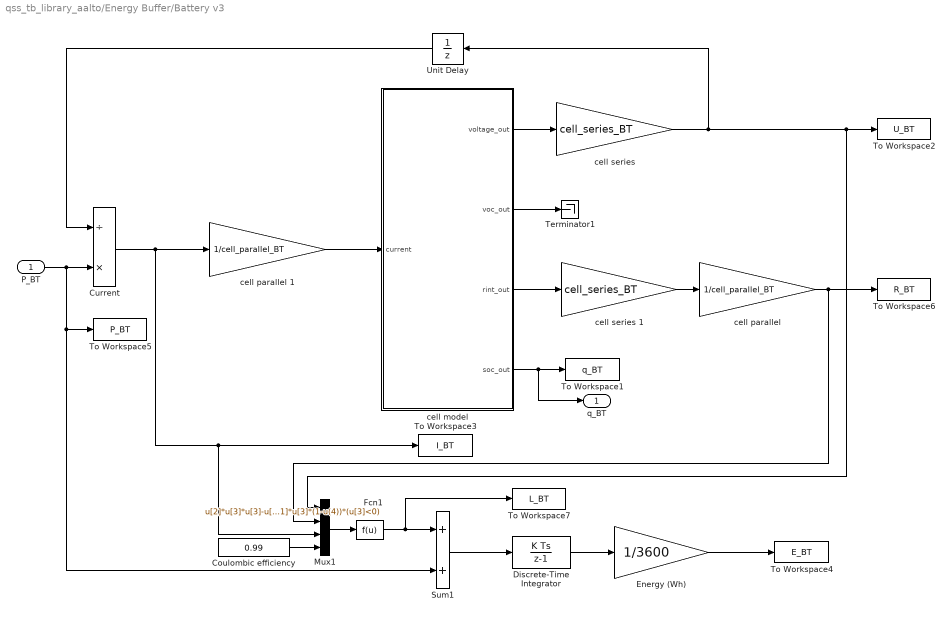
== system qss_tb_library_aalto/Energy Buffer/Battery v3 ==
  P_BT : Inport
  Coulombic efficiency : Constant  Value=0.99
  Current : Product  Inputs=/*  RndMeth=Zero
  Discrete-Time Integrator : DiscreteIntegrator  ICPrevOutput=DiscIntNeverNeededParam  ICPrevScaledInput=DiscIntNeverNeededParam
  Energy (Wh) : Gain  Gain=1/3600
  Fcn1 : Fcn  Expr=u[2]*u[3]*u[3]-u[1]*u[3]*(1-u(4))*(u[3]<0)
  Mux1 : Mux
  Sum1 : Sum  SaturateOnIntegerOverflow=on  InputSameDT=on  OutDataTypeStr=Inherit: Same as first input
  Terminator1 : Terminator
  To Workspace1 : ToWorkspace  VariableName=q_BT  SampleTime=-1
  To Workspace2 : ToWorkspace  VariableName=U_BT  SampleTime=-1
  To Workspace3 : ToWorkspace  VariableName=I_BT  SampleTime=-1
  To Workspace4 : ToWorkspace  VariableName=E_BT  SampleTime=-1
  To Workspace5 : ToWorkspace  VariableName=P_BT  SampleTime=-1
  To Workspace6 : ToWorkspace  VariableName=R_BT  SampleTime=-1
  To Workspace7 : ToWorkspace  VariableName=L_BT  SampleTime=-1
  Unit Delay : UnitDelay  InitialCondition=cell_series_BT*max(voc_map_BT)  SampleTime=-1
  cell model : Subsystem
  cell parallel : Gain  Gain=1/cell_parallel_BT
  cell parallel 1 : Gain  Gain=1/cell_parallel_BT
  "cell series " : Gain  Gain=cell_series_BT
  cell series 1 : Gain  Gain=cell_series_BT
  q_BT : Outport  InitialOutput=0
  wires:
  Coulombic efficiency/1 -> Mux1/4
  Mux1/1 -> Fcn1/1
  Energy (Wh)/1 -> To Workspace4/1
  Sum1/1 -> Discrete-Time Integrator/1
  Fcn1/1 -> To Workspace7/1, Sum1/1
  Discrete-Time Integrator/1 -> Energy (Wh)/1
  cell parallel 1/1 -> cell model/1(current)
  cell parallel/1 -> Mux1/2, To Workspace6/1
  cell model/4(soc_out) -> q_BT/1, To Workspace1/1
  Current/1 -> Mux1/3, To Workspace3/1, cell parallel 1/1
  Unit Delay/1 -> Current/1
  cell model/2(voc_out) -> Terminator1/1
  P_BT/1 -> Sum1/2, To Workspace5/1, Current/2
  cell series 1/1 -> cell parallel/1
  cell model/3(rint_out) -> cell series 1/1
  "cell series "/1 -> Mux1/1, To Workspace2/1, Unit Delay/1
  cell model/1(voltage_out) -> "cell series "/1

== system qss_tb_library_aalto/Energy Buffer/Supercapacitor ==
  P_SC : Inport
  Fcn : Fcn  Expr=(-u[2]/C_SC+sqrt(u[2]^2/C_SC^2-4*R_SC*u[1]))/(2*R_SC)
  Gain : Gain  Gain=1/C_SC  SaturateOnIntegerOverflow=on  OutDataTypeStr=Inherit: Same as input  ParamDataTypeStr=Inherit: Same as input
  Gain1 : Gain  Gain=h  SaturateOnIntegerOverflow=on  OutDataTypeStr=Inherit: Same as input  ParamDataTypeStr=Inherit: Same as input
  Mux : Mux  Inputs=2
  SC charge : UnitDelay  InitialCondition=Q_SC_IC  SampleTime=h
  Sum3 : Sum  SaturateOnIntegerOverflow=on  InputSameDT=on  OutDataTypeStr=Inherit: Same as first input
  Supervision supercap : Subsystem
  To Workspace1 : ToWorkspace  VariableName=I_SC  SampleTime=1
  To Workspace2 : ToWorkspace  VariableName=U_SC  SampleTime=1
  To Workspace3 : ToWorkspace  VariableName=Q_SC  SampleTime=1
  To Workspace4 : ToWorkspace  VariableName=P_SC  SampleTime=1
  U_SC : Outport  InitialOutput=0
  wires:
  P_SC/1 -> Supervision supercap/2(P_SC), Mux/1, To Workspace4/1
  Gain/1 -> To Workspace2/1, U_SC/1
  Fcn/1 -> To Workspace1/1, Gain1/1
  SC charge/1 -> To Workspace3/1, Supervision supercap/1(Q_SC), Mux/2, Gain/1, Sum3/2
  Sum3/1 -> SC charge/1
  Mux/1 -> Fcn/1
  Gain1/1 -> Sum3/1
